simulink model "sac"  (R2015a)
settings: Solver=ode45  StartTime=0.0  StopTime=20  RelTol=1e-3
values from neighbouring files (symbols this model uses):
  a = 100    [sac_params.m]
  am = (1/Jm)*(Dm + Kt*Kb/Ra)    (= 1.70833333333)    [sac_params.m]
  K = 1    [sac_params.m]
  K1 = 100    [sac_params.m]
  Kg = N1/N2    (= 0.1)    [sac_params.m]
  Km = Kt/(Ra*Jm)    (= 2.08333333333)    [sac_params.m]
  Kpot = (2*V)/(n*2*pi)    (= 0.318309886184)    [sac_params.m]
settings Model: Creator=eechris  LastModifiedBy=c.p.jobling
settings DebuggingCC: UnderspecifiedInitializationDetection=Classic  MergeDetectMultiDrivingBlocksExec=none  SolverPrmCheckMsg=warning

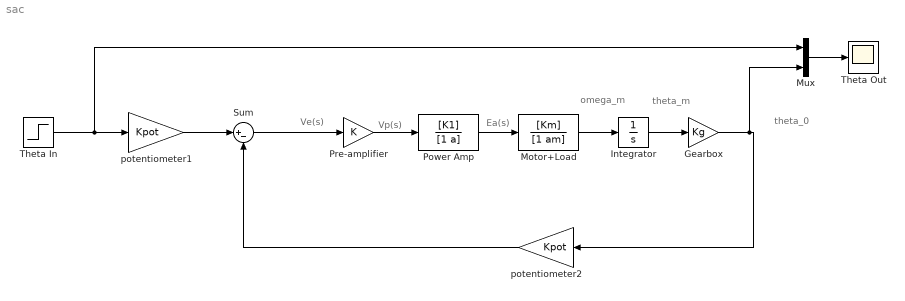
== system sac ==
  note: omega_m
  note: Ea(s)
  note: Vp(s)
  note: Ve(s)
  note: theta_0
  note: theta_m
  Gearbox : Gain  Gain=Kg
  Integrator : Integrator
  Motor+Load : TransferFcn  Numerator=[Km]  Denominator=[1 am]
  Mux : Mux  Inputs=2
  Power Amp : TransferFcn  Numerator=[K1]  Denominator=[1 a]
  Pre-amplifier : Gain  Gain=K
  Sum : Sum  Inputs=|+-
  Theta In : Step  SampleTime=0
  Theta Out : Scope
      settings: YMin=0  YMax=1
  potentiometer1 : Gain  Gain=Kpot
  potentiometer2 : Gain  Gain=Kpot
  wires:
  Integrator/1 -> Gearbox/1
  Power Amp/1 -> Motor+Load/1
  Motor+Load/1 -> Integrator/1
  Gearbox/1 -> Mux/2, potentiometer2/1
  potentiometer1/1 -> Sum/1
  Sum/1 -> Pre-amplifier/1
  potentiometer2/1 -> Sum/2
  Mux/1 -> Theta Out/1
  Theta In/1 -> Mux/1, potentiometer1/1
  Pre-amplifier/1 -> Power Amp/1
